simulink model "Open_Loop"  (R2024a)
settings: Solver=ode45  StartTime=0.0  StopTime=tf  MaxStep=0.005  RelTol=1e-6  EnableMultiTasking=on
values from neighbouring files (symbols this model uses):
  cs = 2e3    (= 2000)    [equilibria.m]    (also in main_v2.m; quarterCarStateJacobianFcn.m; quarterCarStates.m; single_sim_open_loop.m)
  epsilon = 30    [calculus_of_L.m]    (also in equilibria.m = 20; main_v2.m; single_sim_open_loop.m)
  g = 9.81    [calculus_of_L.m]    (also in equilibria.m; main_v2.m; quarterCarStates.m; single_sim_open_loop.m)
  ks = 20e3    (= 20000)    [calculus_of_L.m]    (also in equilibria.m; main_v2.m; single_sim_open_loop.m)
  ku = 2.5e5    (= 250000)    [calculus_of_L.m]    (also in equilibria.m; main_v2.m; single_sim_open_loop.m)
  Ls = (ms*g/ks)-(zu_bar-zs_bar)-epsilon*(zu_bar-zs_bar)^3    (= 0.3948885)    [calculus_of_L.m]    (also in equilibria.m = 0.4; main_v2.m = 0.4; quarterCarStateJacobianFcn.m = 0.4; quarterCarStates.m = 0.4)
  Lu = (ks*(zu_bar-zs_bar)+(ks*epsilon*(zu_bar-zs_bar)^3)+ks*Ls+ku*zu_bar+mu*g)/ku    (= 0.34460348)    [calculus_of_L.m]    (also in equilibria.m = 0.34; main_v2.m = 0.34; quarterCarStateJacobianFcn.m = 0.34; quarterCarStates.m = 0.34)
  mass_person = 0    [main_v2.m]
  mass_wheel = 0    [main_v2.m]
  ms = 577    [calculus_of_L.m]    (also in equilibria.m; main_v2.m; quarterCarStateJacobianFcn.m; quarterCarStates.m)
  mu = 50    [calculus_of_L.m]    (also in equilibria.m; main_v2.m; quarterCarStateJacobianFcn.m; quarterCarStates.m)
  roadType = input('Enter choice (1-2): ')    [main_v2.m]
  sat = 6000    [main_v2.m]
  sosp = 1    [main_v2.m]
  ts = 0.01    [main_v2.m]    (also in off_road_profile.mat; road_profile_bump.mat)
  uncertainty = 0    [main_v2.m]
  x0 = [0.001, -0.001, 0.001, -0.001]    [main_v2.m]    (also in single_sim_open_loop.m = xA + alpha * v)
  x_eq = [0.408, 0.315, 0, 0]    [main_v2.m]
libraries: simulink x2
settings Model: Creator=arsen  LastModifiedBy=arsen
settings DataIOCC: LimitDataPoints=on  MaxDataPoints=10000  SaveFormat=Array  SignalLoggingSaveFormat=ModelDataLogs  ReturnWorkspaceOutputs=off
settings OptimizationCC: InitFltsAndDblsToZero=on  LifeSpan=inf
settings DebuggingCC: SaveWithParameterizedLinksMsg=none  UnderspecifiedInitializationDetection=Classic  MergeDetectMultiDrivingBlocksExec=none  SignalResolutionControl=TryResolveAllWithWarning  SolverPrmCheckMsg=warning  MultiTaskDSMMsg=warning  MultiTaskCondExecSysMsg=none  FcnCallInpInsideContextMsg=warning  UnconnectedInputMsg=warning  UnconnectedOutputMsg=warning  UnconnectedLineMsg=warning  SFUnexpectedBacktrackingDiag=warning  SFNoUnconditionalDefaultTransitionDiag=warning  SFExecutionAtInitializationDiag=none  ArithmeticOperatorsInVariantConditions=warning
settings HardwareCC: ProdBitPerPointer=32  ProdBitPerSizeT=32  ProdBitPerPtrDiffT=32  ProdLargestAtomicFloat=None  ProdIntDivRoundTo=Undefined  ProdEndianess=Unspecified  ProdWordSize=32  ProdHWDeviceType=32-bit Generic
settings ModelReferenceCC: PropagateSignalLabelsOutOfModel=off
settings RTWCC: GPUComputeCapability=3.5
settings CodeAppCC: StateflowObjectComments=on
settings GRTTargetCC: TargetFcnLib=ansi_tfl_tmw.mat  TargetLangStandard=C89/C90 (ANSI)  CombineOutputUpdateFcns=off  GRTInterface=on
settings ConfigComp: CovMetricSettings=dw  CovSaveCumulativeToWorkspaceVar=on  CovSaveSingleToWorkspaceVar=on

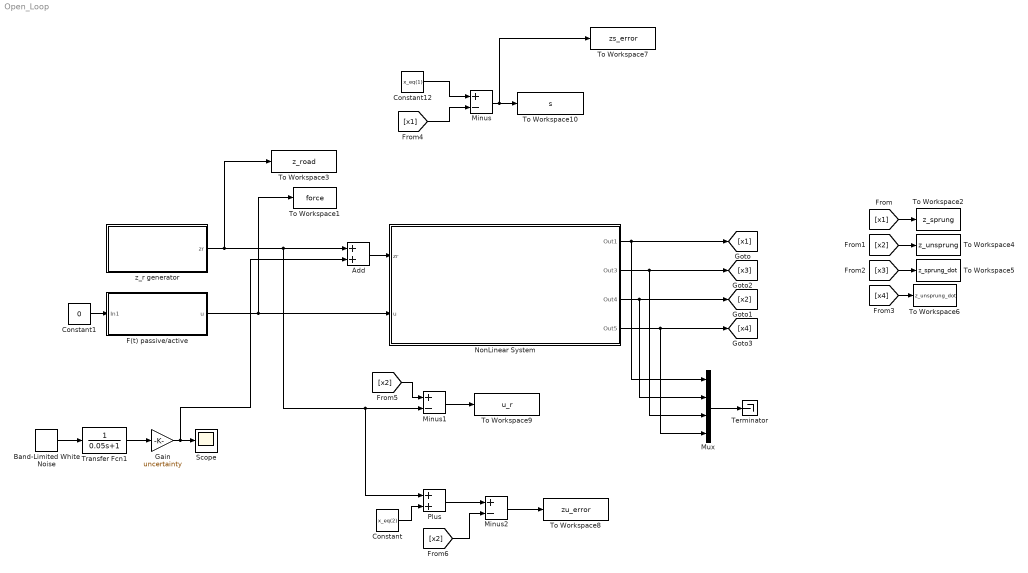
== system Open_Loop ==
  Add : Sum
  Band-Limited White Noise : simulink/Sources/Band-Limited White Noise  Cov=[1]  Ts=ts  seed=[23341]
  Constant : Constant  Value=x_eq(2)
  Constant1 : Constant  Value=0
  Constant12 : Constant  Value=x_eq(1)
  F(t) passive/active : Subsystem
  Gain : Gain  Gain=uncertainty
  Minus : Sum  Inputs=+-
  Minus1 : Sum  Inputs=+-
  Minus2 : Sum  Inputs=+-
  Mux : Mux
  NonLinear System : Subsystem
  Plus : Sum
  Scope : Scope
  Terminator : Terminator
  To Workspace1 : ToWorkspace  VariableName=force  SampleTime=-1
  To Workspace10 : ToWorkspace  VariableName=s  SampleTime=-1
  To Workspace2 : ToWorkspace  VariableName=z_sprung  SampleTime=-1
  To Workspace3 : ToWorkspace  VariableName=z_road  SampleTime=-1
  To Workspace4 : ToWorkspace  VariableName=z_unsprung  SampleTime=-1
  To Workspace5 : ToWorkspace  VariableName=z_sprung_dot  SampleTime=-1
  To Workspace6 : ToWorkspace  VariableName=z_unsprung_dot  SampleTime=-1
  To Workspace7 : ToWorkspace  VariableName=zs_error  SampleTime=-1
  To Workspace8 : ToWorkspace  VariableName=zu_error  SampleTime=-1
  To Workspace9 : ToWorkspace  VariableName=u_r  SampleTime=-1
  Transfer Fcn1 : TransferFcn  Denominator=[0.05 1]
  z_r generator : Subsystem
  wires:
  F(t) passive/active/1(u) -> To Workspace1/1, NonLinear System/2(u)
  z_r generator/1(zr) -> Plus/1, Minus1/2, Add/1, To Workspace3/1
  Minus/1 -> To Workspace10/1, To Workspace7/1
  Minus1/1 -> To Workspace9/1
  Constant/1 -> Plus/2
  Minus2/1 -> To Workspace8/1
  Constant12/1 -> Minus/1
  Plus/1 -> Minus2/1
  NonLinear System/1(Out1) -> Mux/1, [x1]
  [x1] -> To Workspace2/1
  NonLinear System/3(Out4) -> Mux/2, [x2]
  NonLinear System/2(Out3) -> Mux/3, [x3]
  [x3] -> To Workspace5/1
  [x2] -> To Workspace4/1
  NonLinear System/4(Out5) -> Mux/4, [x4]
  [x4] -> To Workspace6/1
  [x1] -> Minus/2
  [x2] -> Minus1/1
  [x2] -> Minus2/2
  Mux/1 -> Terminator/1
  Constant1/1 -> F(t) passive/active/1(In1)
  Transfer Fcn1/1 -> Gain/1
  Gain/1 -> Add/2, Scope/1
  Band-Limited White Noise/1 -> Transfer Fcn1/1
  Add/1 -> NonLinear System/1(zr)

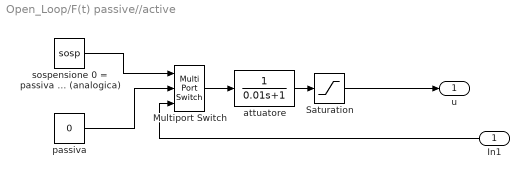
== system Open_Loop/F(t) passive//active ==
  In1 : Inport
  Multiport Switch : MultiPortSwitch  DataPortOrder=Zero-based contiguous  Inputs=2  zeroidx=on  SaturateOnIntegerOverflow=off  InputSameDT=off
  Saturation : Saturate  UpperLimit=sat  LowerLimit=-sat
  attuatore : TransferFcn  Numerator=1  Denominator=[0.01 1]
  "passiva " : Constant  Value=0
  sospensione 0 = passiva 1 = attiva (analogica) : Constant  Value=sosp
  u : Outport
  wires:
  sospensione 0 = passiva 1 = attiva (analogica)/1 -> Multiport Switch/1
  Multiport Switch/1 -> attuatore/1
  attuatore/1 -> Saturation/1
  "passiva "/1 -> Multiport Switch/2
  In1/1 -> Multiport Switch/3
  Saturation/1 -> u/1

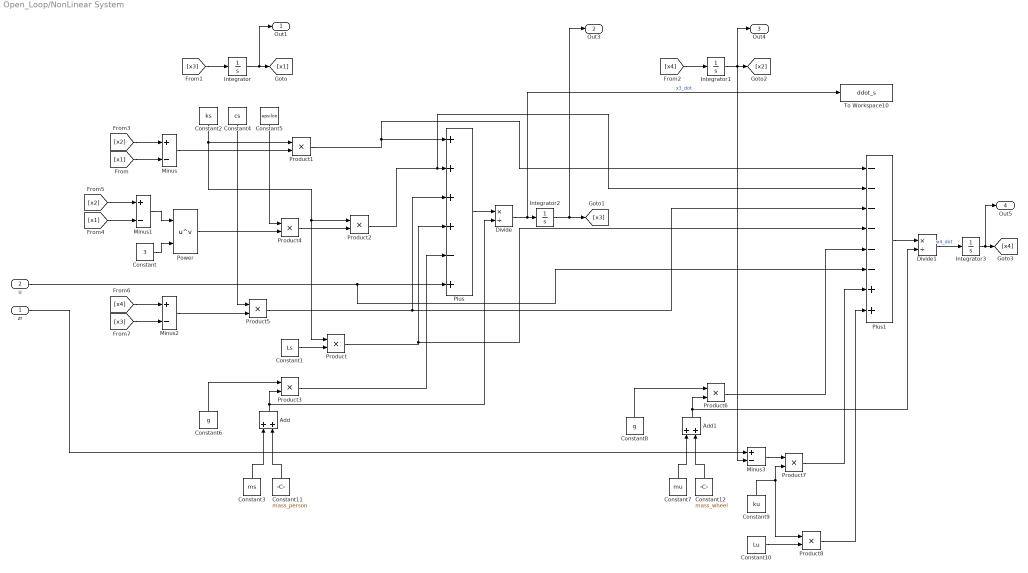
== system Open_Loop/NonLinear System ==
  zr : Inport
  u : Inport  Port=2
  Add : Sum
  Add1 : Sum
  Constant : Constant  Value=3
  Constant1 : Constant  Value=Ls
  Constant10 : Constant  Value=Lu
  Constant11 : Constant  Value=mass_person
  Constant12 : Constant  Value=mass_wheel
  Constant2 : Constant  Value=ks
  Constant3 : Constant  Value=ms
  Constant4 : Constant  Value=cs
  Constant5 : Constant  Value=epsilon
  Constant6 : Constant  Value=g
  Constant7 : Constant  Value=mu
  Constant8 : Constant  Value=g
  Constant9 : Constant  Value=ku
  Divide : Product  Inputs=*/  RndMeth=Zero  SaturateOnIntegerOverflow=on
  Divide1 : Product  Inputs=*/  RndMeth=Zero  SaturateOnIntegerOverflow=on
  Integrator : Integrator  InitialCondition=x0(1)+x_eq(1)
  Integrator1 : Integrator  InitialCondition=x0(2)+x_eq(2)
  Integrator2 : Integrator  InitialCondition=x0(3)
  Integrator3 : Integrator  InitialCondition=x0(4)
  Minus{,1..3} (4 alike) : Sum  Inputs=+-
  Plus : Sum  Inputs=++++-+
  Plus1 : Sum  Inputs=------++
  Power : Math  Operator=pow
  Product{,1..8} (9 alike) : Product
  To Workspace10 : ToWorkspace  VariableName=ddot_s  SampleTime=-1
  Out1 : Outport
  Out3 : Outport  Port=2
  Out4 : Outport  Port=3
  Out5 : Outport  Port=4
  wires:
  Plus/1 -> Divide/1
  Product4/1 -> Product2/2
  Divide/1 -> To Workspace10/1, Integrator2/1  "x3_dot"
  Divide1/1 -> Integrator3/1  "x4_dot"
  Product8/1 -> Plus1/8
  Product6/1 -> Plus1/5
  Power/1 -> Product4/2
  [x2] -> Minus/1
  [x2] -> Minus1/1
  Minus/1 -> Product1/2
  Product5/1 -> Plus1/3, Plus/3
  Constant5/1 -> Product4/1
  Constant8/1 -> Product6/1
  [x4] -> Minus2/1
  [x4] -> Integrator1/1
  Product1/1 -> Plus1/1, Plus/1
  Constant1/1 -> Product/2
  Constant2/1 -> Product2/1, Product/1, Product1/1
  Minus2/1 -> Product5/2
  Constant9/1 -> Product8/1, Product7/2
  Integrator/1 -> Out1/1, [x1]
  Product/1 -> Plus/4, Plus1/4
  zr/1 -> Minus3/1
  Constant/1 -> Power/2
  Constant6/1 -> Product3/1
  Integrator3/1 -> Out5/1, [x4]
  [x1] -> Minus1/2
  [x1] -> Minus/2
  Integrator2/1 -> Out3/1, [x3]
  Integrator1/1 -> Minus3/2, Out4/1, [x2]
  Product3/1 -> Plus/5
  [x3] -> Integrator/1
  Constant4/1 -> Product5/1
  u/1 -> Plus1/6, Plus/6
  Minus1/1 -> Power/1
  Product7/1 -> Plus1/7
  [x3] -> Minus2/2
  Product2/1 -> Plus1/2, Plus/2
  Plus1/1 -> Divide1/1
  Constant10/1 -> Product8/2
  Minus3/1 -> Product7/1
  Constant11/1 -> Add/2
  Constant3/1 -> Add/1
  Add/1 -> Divide/2, Product3/2
  Add1/1 -> Divide1/2, Product6/2
  Constant12/1 -> Add1/2
  Constant7/1 -> Add1/1

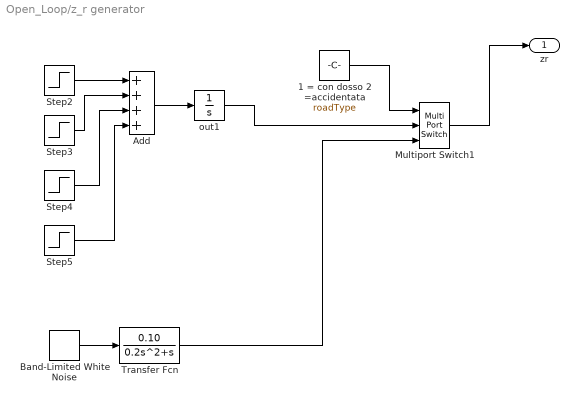
== system Open_Loop/z_r generator ==
  1 = con dosso 2 =accidentata : Constant  Value=roadType
  Add : Sum  Inputs=++++
  Band-Limited White Noise : simulink/Sources/Band-Limited White Noise  Cov=[0.1]  Ts=ts  seed=[23341]
  Multiport Switch1 : MultiPortSwitch  Inputs=2  SaturateOnIntegerOverflow=off  InputSameDT=off
  Step2 : Step  After=0.5/6  SampleTime=0
  Step3 : Step  Time=1.5  After=-0.5/6  SampleTime=0
  Step4 : Step  Time=2.5  After=-0.5/6  SampleTime=0
  Step5 : Step  Time=3  After=0.5/6  SampleTime=0
  Transfer Fcn : TransferFcn  Numerator=[0.10]  Denominator=[0.2 1 0]
  out1 : Integrator  InitialCondition=[0]
  zr : Outport
  wires:
  Step2/1 -> Add/1
  Multiport Switch1/1 -> zr/1
  Step4/1 -> Add/3
  Band-Limited White Noise/1 -> Transfer Fcn/1
  1 = con dosso 2 =accidentata/1 -> Multiport Switch1/1
  Step5/1 -> Add/4
  Step3/1 -> Add/2
  Add/1 -> out1/1
  out1/1 -> Multiport Switch1/2
  Transfer Fcn/1 -> Multiport Switch1/3
